simulink model "smithPredictorExample1Simulink"  (R2023b)
settings: Solver=VariableStepAuto  StartTime=0.0  StopTime=Tsim  RelTol=1e-3
values from neighbouring files (symbols this model uses):
  Cz = c2d(C1C,Ts)    [smithPredictorExample1Code.m]
  finalDisturbance1Value = 0.8    [smithPredictorExample1Code.m]
  finalDisturbance2Value = 0.8    [smithPredictorExample1Code.m]
  finalReference1Value = 1    [smithPredictorExample1Code.m]
  finalReference2Value = 1    [smithPredictorExample1Code.m]
  initialDisturbance1Value = 0.1    [smithPredictorExample1Code.m]
  initialDisturbance2Value = 0.1    [smithPredictorExample1Code.m]
  initialReference1Value = 0    [smithPredictorExample1Code.m]
  initialReference2Value = 0    [smithPredictorExample1Code.m]
  Pz = Gz*Lz    [smithPredictorExample1Code.m]
  Tref1 = 0    [smithPredictorExample1Code.m]
  Tref2 = 15    [smithPredictorExample1Code.m]
  Ts = 0.03*sU    (= 0.03)    [smithPredictorExample1Code.m]
libraries: cstblocks x10
settings Model: Creator=klysm  LastModifiedBy=klysm

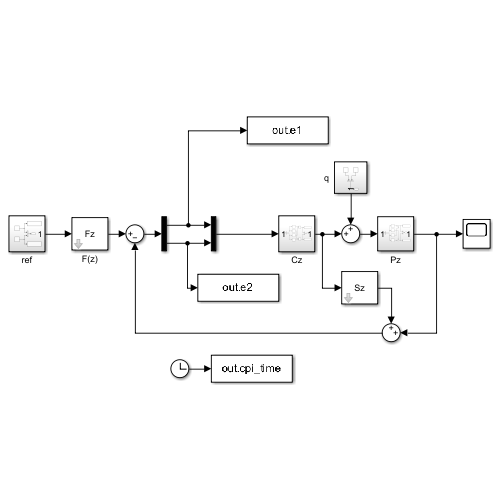
[thumbnail: Simulink's stored preview of the top-level diagram]
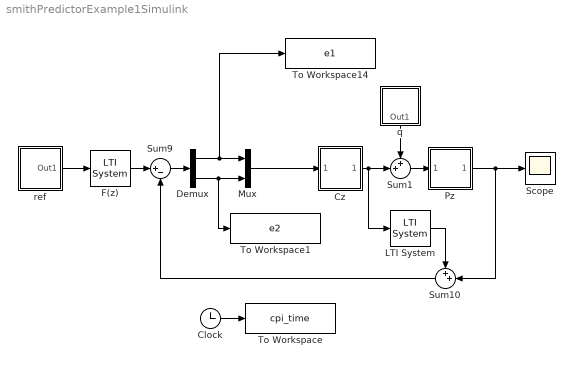
== system smithPredictorExample1Simulink ==
  Clock : Clock
  Cz : Subsystem
  Demux : Demux  Outputs=2
  F(z) : cstblocks/LTI System  sys=Fz  IC=[]  PadeOrder=0
  LTI System : cstblocks/LTI System  sys=Sz  IC=[]  PadeOrder=0
  Mux : Mux  Inputs=2
  Pz : Subsystem
  Scope : Scope
  Sum1 : Sum  Inputs=++|
  Sum10 : Sum  Inputs=++|
  Sum9 : Sum  Inputs=|+-
  To Workspace : ToWorkspace  VariableName=cpi_time  SampleTime=Ts
  To Workspace1 : ToWorkspace  VariableName=e2  SampleTime=Ts
  To Workspace14 : ToWorkspace  VariableName=e1  SampleTime=Ts
  q : Subsystem
  ref : Subsystem
  wires:
  LTI System/1 -> Sum10/1
  Sum1/1 -> Pz/1(In1)
  q/1(Out1) -> Sum1/1
  Mux/1 -> Cz/1(In1)
  Cz/1(Out1) -> Sum1/2, LTI System/1
  Pz/1(Out1) -> Scope/1, Sum10/2
  ref/1(Out1) -> F(z)/1
  Clock/1 -> To Workspace/1
  Sum10/1 -> Sum9/2
  Demux/2 -> To Workspace1/1, Mux/2
  Demux/1 -> To Workspace14/1, Mux/1
  Sum9/1 -> Demux/1
  F(z)/1 -> Sum9/1

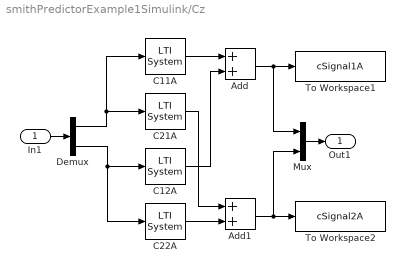
== system smithPredictorExample1Simulink/Cz ==
  In1 : Inport
  Add : Sum
  Add1 : Sum
  C11A : cstblocks/LTI System  sys=Cz(1,1)  IC=[]  PadeOrder=0
  C12A : cstblocks/LTI System  sys=Cz(1,2)  IC=[]  PadeOrder=0
  C21A : cstblocks/LTI System  sys=Cz(2,1)  IC=[]  PadeOrder=0
  C22A : cstblocks/LTI System  sys=Cz(2,2)  IC=[]  PadeOrder=0
  Demux : Demux  Outputs=2
  Mux : Mux  Inputs=2
  To Workspace1 : ToWorkspace  VariableName=cSignal1A  SampleTime=Ts
  To Workspace2 : ToWorkspace  VariableName=cSignal2A  SampleTime=Ts
  Out1 : Outport
  wires:
  Add1/1 -> To Workspace2/1, Mux/2
  C21A/1 -> Add1/1
  C22A/1 -> Add1/2
  C11A/1 -> Add/1
  Add/1 -> To Workspace1/1, Mux/1
  In1/1 -> Demux/1
  Demux/1 -> C11A/1, C21A/1
  C12A/1 -> Add/2
  Demux/2 -> C22A/1, C12A/1
  Mux/1 -> Out1/1

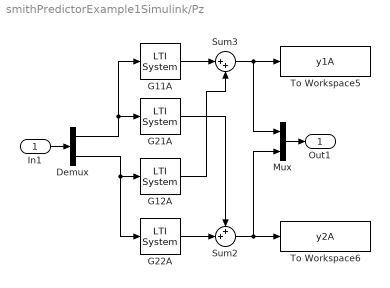
== system smithPredictorExample1Simulink/Pz ==
  In1 : Inport
  Demux : Demux  Outputs=2
  G11A : cstblocks/LTI System  sys=Pz(1,1)  IC=[]  PadeOrder=0
  G12A : cstblocks/LTI System  sys=Pz(1,2)  IC=[]  PadeOrder=0
  G21A : cstblocks/LTI System  sys=Pz(2,1)  IC=[]  PadeOrder=0
  G22A : cstblocks/LTI System  sys=Pz(2,2)  IC=[]  PadeOrder=0
  Mux : Mux  Inputs=2
  Sum2 : Sum  Inputs=++|
  Sum3 : Sum  Inputs=|++
  To Workspace5 : ToWorkspace  VariableName=y1A  SampleTime=Ts
  To Workspace6 : ToWorkspace  VariableName=y2A  SampleTime=Ts
  Out1 : Outport
  wires:
  Sum2/1 -> To Workspace6/1, Mux/2
  G11A/1 -> Sum3/1
  Demux/1 -> G11A/1, G21A/1
  Demux/2 -> G22A/1, G12A/1
  Mux/1 -> Out1/1
  G12A/1 -> Sum3/2
  G22A/1 -> Sum2/2
  G21A/1 -> Sum2/1
  Sum3/1 -> To Workspace5/1, Mux/1
  In1/1 -> Demux/1

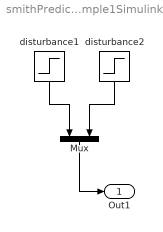
== system smithPredictorExample1Simulink/q ==
  Mux : Mux  Inputs=2
  disturbance1 : Step  Time=Tref1  Before=initialDisturbance1Value  After=finalDisturbance1Value  SampleTime=Ts
  disturbance2 : Step  Time=Tref2  Before=initialDisturbance2Value  After=finalDisturbance2Value  SampleTime=Ts
  Out1 : Outport
  wires:
  disturbance2/1 -> Mux/2
  disturbance1/1 -> Mux/1
  Mux/1 -> Out1/1

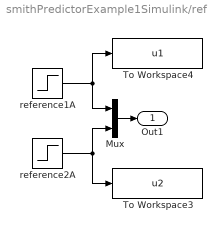
== system smithPredictorExample1Simulink/ref ==
  Mux : Mux  Inputs=2
  To Workspace3 : ToWorkspace  VariableName=u2  SampleTime=Ts
  To Workspace4 : ToWorkspace  VariableName=u1  SampleTime=Ts
  reference1A : Step  Time=Tref1  Before=initialReference1Value  After=finalReference1Value  SampleTime=Ts
  reference2A : Step  Time=Tref2  Before=initialReference2Value  After=finalReference2Value  SampleTime=Ts
  Out1 : Outport
  wires:
  reference1A/1 -> Mux/1, To Workspace4/1
  Mux/1 -> Out1/1
  reference2A/1 -> To Workspace3/1, Mux/2
